simulink model "tb_FFT"  (R2024a)
settings: Solver=FixedStepDiscrete  StartTime=0.0  StopTime=400  RelTol=1e-3
undefined symbols (not defined in the file): F1, F2, FFTLength, Fs, ReadyIn, Reset, TestMode, Threshold
libraries: dsphdlxfrm2 x1, simulink x1
settings Model: DataTypeOverride=Off  Creator=bsingh  LastModifiedBy=bsingh
settings OptimizationCC: BlockReduction=off  ConditionallyExecuteInputs=off  DefaultParameterBehavior=Inlined  InheritOutputTypeSmallerThanSingle=on  OptimizeBlockIOStorage=off  ReuseModelBlockBuffer=off  EnhancedBackFolding=on  PassReuseOutputArgsThreshold=0  OptimizeBlockOrder=speed  DifferentSizesBufferReuse=on
settings DebuggingCC: AlgebraicLoopMsg=error  SingleTaskRateTransMsg=error  ParameterTunabilityLossMsg=error
settings HardwareCC: ProdBitPerPointer=32  ProdBitPerSizeT=32  ProdBitPerPtrDiffT=32  ProdLargestAtomicFloat=None  ProdIntDivRoundTo=Undefined  ProdEndianess=Unspecified  ProdWordSize=32  ProdHWDeviceType=ASIC/FPGA->ASIC/FPGA  TargetBitPerPointer=64  TargetBitPerSizeT=64  TargetBitPerPtrDiffT=64  TargetLongLongMode=on  TargetIntDivRoundTo=Zero  TargetEndianess=LittleEndian  TargetWordSize=64  TargetHWDeviceType=Generic->Custom  ProdEqTarget=off
settings SFSimCC: MATLABDynamicMemAllocThreshold=1024
settings RTWCC: Description=SystemVerilog DPI Component Generator  SystemTargetFile=systemverilog_dpi_grt.tlc  TemplateMakefile=systemverilog_dpi_grt_default_tmf  GPUComputeCapability=3.5
settings CodeAppCC: ForceParamTrailComments=on  MaxIdLength=256  OperatorAnnotations=on
settings DPIGRTTargetCC: TargetFcnLib=ansi_tfl_table_tmw.mat  GenFloatMathFcnCalls=NOT IN USE  TargetLangStandard=C89/C90 (ANSI)  CodeReplacementLibrary=None  UtilityFuncGeneration=Auto  MultiwordTypeDef=System defined  MultiwordLength=2048  DynamicStringBufferSize=256  GenerateFullHeader=on  InferredTypesCompatibility=off  GenerateSampleERTMain=off  GenerateTestInterfaces=off  ModelReferenceCompliant=on  ParMdlRefBuildCompliant=on  CompOptLevelCompliant=off  ConcurrentExecutionCompliant=off  IncludeMdlTerminateFcn=on  CombineOutputUpdateFcns=off  CombineSignalStateStructs=on  GroupInternalDataByFunction=off  SuppressErrorStatus=off  IncludeFileDelimiter=Auto  ERTCustomFileBanners=off  SupportAbsoluteTime=on  LogVarNameModifier=rt_  MatFileLogging=off  CodeInterfacePackaging=Reusable function  PurelyIntegerCode=off  SupportNonFinite=on  SupportComplex=on  SupportContinuousTime=on  SupportNonInlinedSFcns=on  RemoveDisableFunc=off  RemoveResetFunc=off  SupportVariableSizeSignals=off  ParenthesesLevel=Nominal  CastingMode=Nominal  MATLABClassNameForMDSCustomization=Simulink.SoftwareTarget.TargetSpecificTriggerConfigurationBase  ModelStepFunctionPrototypeControlCompliant=off  CPPClassGenCompliant=off  AutosarCompliant=off  MDXCompliant=off  GRTInterface=off  GenerateAllocFcn=on  UseToolchainInfoCompliant=on  GenerateSharedConstants=on  CoderGroups=[]  AccessMethods=[]  LookupTableObjectStructAxisOrder=1,2,3,4,...  LUTObjectStructOrderExplicitValues=Size,Breakpoints,Table  LUTObjectStructOrderEvenSpacing=Size,Breakpoints,Table  ArrayLayout=Column-major  UnsupportedSFcnMsg=error  ERTHeaderFileRootName=$R$E  ERTSourceFileRootName=$R$E  ERTDataFileRootName=$R_data  InstructionSetFMA=off  OptimizeReductions=off  LogToMDFFile=off  DPICustomizeSystemVerilogCode=off  DPISystemVerilogTemplate=svdpi_event.vgt  DPIReportRunTimeError=off  DPIRunTimeErrorSeverity=Fatal  DPIScalarizePorts=off  DPIGenerateTestBench=off  DPITestBenchSimulator=Mentor Graphics Questasim  DPITestPointAccessFcnInterface=None  DPIFixedPointDataType=CompatibleCType  DPIPortConnection=Port list  DPICompositeDataType=Structure  DPIComponentTemplateType=Sequential  ExtMode=off  ExtModeStaticAlloc=off  ExtModeTesting=off  ExtModeStaticAllocSize=1000000  ExtModeTransport=0  ExtModeMexFile=ext_comm  RTWCAPISignals=on  RTWCAPIParams=off  RTWCAPIStates=off  RTWCAPIRootIO=off  GenerateASAP2=off  MultiInstanceErrorCode=Error

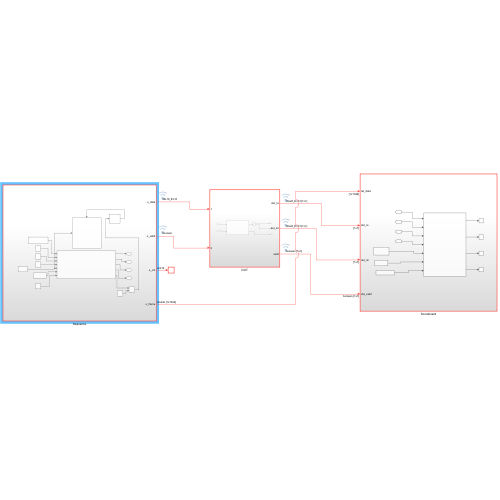
[thumbnail: Simulink's stored preview of the top-level diagram]
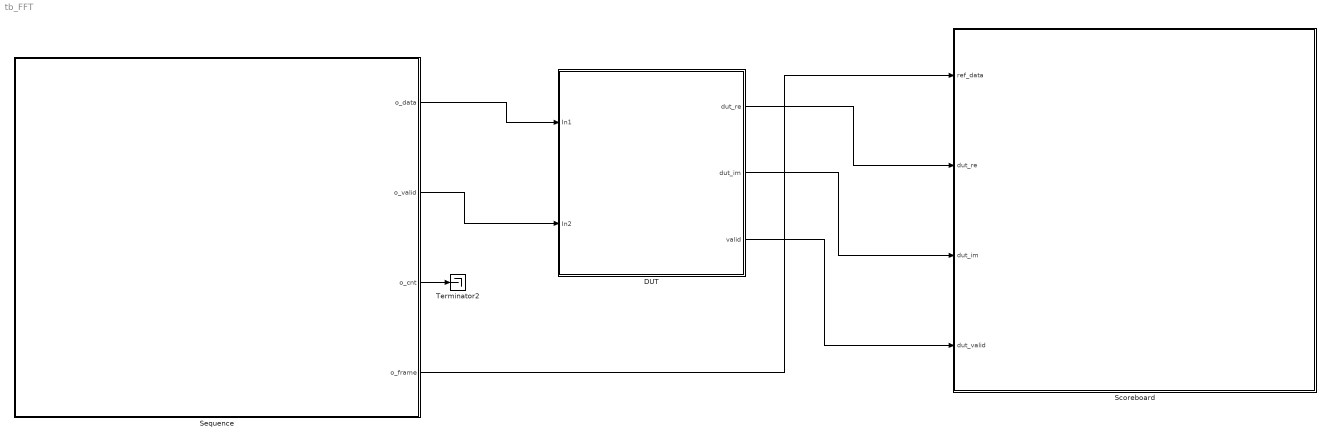
== system tb_FFT ==
  DUT : Subsystem
  Scoreboard : Subsystem
  Sequence : Subsystem
  Terminator2 : Terminator
  wires:
  Sequence/4(o_frame) -> Scoreboard/1(ref_data)
  Sequence/3(o_cnt) -> Terminator2/1
  Sequence/2(o_valid) -> DUT/2(In2)
  Sequence/1(o_data) -> DUT/1(In1)
  DUT/1(dut_re) -> Scoreboard/2(dut_re)
  DUT/2(dut_im) -> Scoreboard/3(dut_im)
  DUT/3(valid) -> Scoreboard/4(dut_valid)

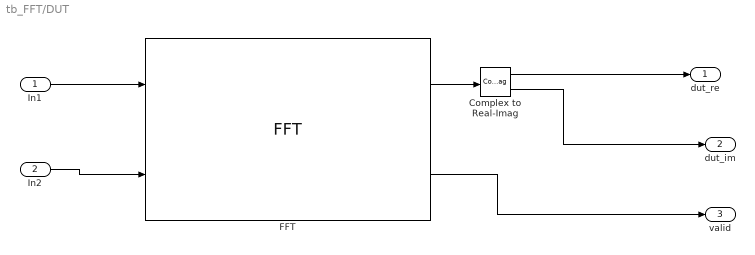
== system tb_FFT/DUT ==
  In1 : Inport
  In2 : Inport  Port=2
  Complex to Real-Imag : ComplexToRealImag
  FFT : dsphdlxfrm2/FFT  Architecture=Streaming Radix 2^2  FFTLengthSource=Property  FFTLength=DUT_FFTLength  FFTLengthMax=1024  ComplexMultiplication=Use 4 multipliers and 2 adders  BitReversedOutput=off  BitReversedInput=off  Normalize=off  SimulateUsing=Code generation  RoundingMethod=Floor  ResetInputPort=off  StartOutputPort=off  EndOutputPort=off
  dut_re : Outport
  dut_im : Outport  Port=2
  valid : Outport  Port=3
  wires:
  FFT/1 -> Complex to Real-Imag/1
  Complex to Real-Imag/2 -> dut_im/1
  Complex to Real-Imag/1 -> dut_re/1
  FFT/2 -> valid/1
  In1/1 -> FFT/1
  In2/1 -> FFT/2

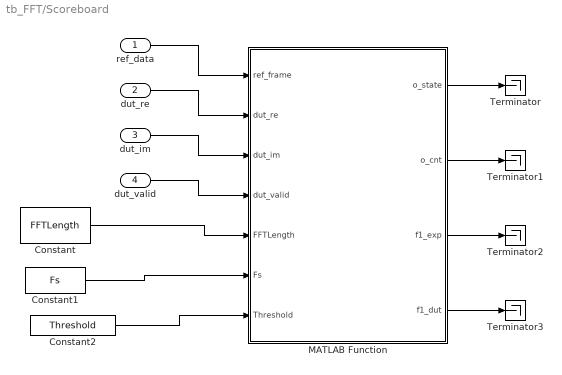
== system tb_FFT/Scoreboard ==
  ref_data : Inport
  dut_re : Inport  Port=2
  dut_im : Inport  Port=3
  dut_valid : Inport  Port=4  OutDataTypeStr=boolean
  Constant : Constant  Value=FFTLength  OutDataTypeStr=Inherit: Inherit via back propagation
  Constant1 : Constant  Value=Fs
  Constant2 : Constant  Value=Threshold
  MATLAB Function : MATLAB Function  TreatAsAtomicUnit=on
  Terminator{,1..3} (4 alike) : Terminator
  wires:
  ref_data/1 -> MATLAB Function/1(ref_frame)
  dut_re/1 -> MATLAB Function/2(dut_re)
  Constant1/1 -> MATLAB Function/6(Fs)
  Constant/1 -> MATLAB Function/5(FFTLength)
  dut_im/1 -> MATLAB Function/3(dut_im)
  dut_valid/1 -> MATLAB Function/4(dut_valid)
  Constant2/1 -> MATLAB Function/7(Threshold)
  MATLAB Function/1(o_state) -> Terminator/1
  MATLAB Function/2(o_cnt) -> Terminator1/1
  MATLAB Function/3(f1_exp) -> Terminator2/1
  MATLAB Function/4(f1_dut) -> Terminator3/1

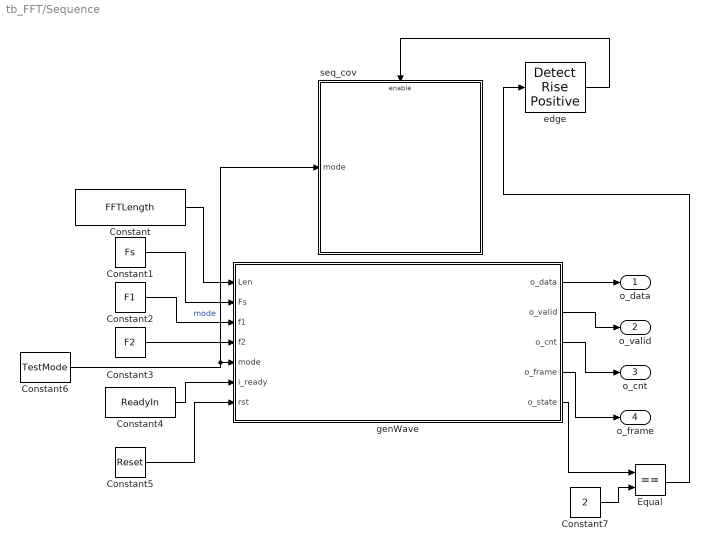
== system tb_FFT/Sequence ==
  Constant : Constant  Value=FFTLength
  Constant1 : Constant  Value=Fs  SampleTime=1e-1
  Constant2 : Constant  Value=F1
  Constant3 : Constant  Value=F2
  Constant4 : Constant  Value=ReadyIn
  Constant5 : Constant  Value=Reset
  Constant6 : Constant  Value=TestMode
  Constant7 : Constant  Value=2
  Equal : RelationalOperator  Operator===  OutDataTypeStr=boolean  RndMeth=Simplest  InputSameDT=off
  edge : simulink/Logic and Bit Operations/Detect Rise Positive  vinit=0  OutDataTypeStr=boolean
  genWave : MATLAB Function  TreatAsAtomicUnit=on
  seq_cov : Subsystem
  o_data : Outport
  o_valid : Outport  Port=2
  o_cnt : Outport  Port=3
  o_frame : Outport  Port=4
  wires:
  Constant5/1 -> genWave/7(rst)
  Constant4/1 -> genWave/6(i_ready)
  genWave/3(o_cnt) -> o_cnt/1
  Constant3/1 -> genWave/4(f2)
  Constant2/1 -> genWave/3(f1)
  Constant1/1 -> genWave/2(Fs)
  Constant/1 -> genWave/1(Len)
  genWave/1(o_data) -> o_data/1
  genWave/4(o_frame) -> o_frame/1
  genWave/2(o_valid) -> o_valid/1
  genWave/5(o_state) -> Equal/1
  Constant6/1 -> seq_cov/1(mode), genWave/5(mode)  "mode"
  Constant7/1 -> Equal/2
  Equal/1 -> edge/1
  edge/1 -> seq_cov/Enable

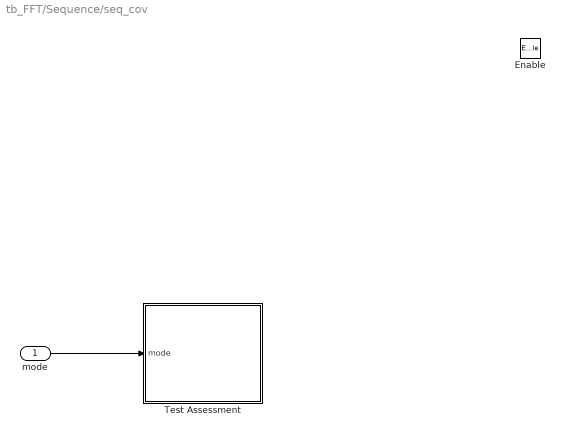
== system tb_FFT/Sequence/seq_cov ==
  mode : Inport
  Enable : EnablePort
  Test Assessment : Test Sequence  TreatAsAtomicUnit=on
  wires:
  mode/1 -> Test Assessment/1(mode)

== matlab function tb_FFT/Scoreboard/MATLAB Function ==
  data: ref_frame input; dut_re input; dut_im input; dut_valid input; FFTLength input; Fs input; o_state output; o_cnt output; Threshold input; f1_exp output; f1_dut output
function [o_state,o_cnt,f1_exp,f1_dut] = scbd(ref_frame,dut_re, dut_im,dut_valid,FFTLength, Fs,Threshold)

[o_state,o_cnt,f1_exp,f1_dut] = fftchecker(ref_frame,dut_re,dut_im,dut_valid,double(FFTLength),double(Fs),Threshold);

end

== matlab function tb_FFT/Sequence/genWave ==
  data: Len input; o_data output; Fs input; f1 input; f2 input; mode input; i_ready input; rst input; o_valid output; o_cnt output; o_frame output; o_state output
function [o_data,o_valid,o_cnt,o_frame,o_state] = genWave(Len,Fs,f1,f2,mode,i_ready,rst)%#codegen

[o_data,o_valid,o_cnt,o_frame,o_state] = genframe2Sample(Len, Fs,f1,f2,mode,i_ready,rst);

end

== stateflow chart tb_FFT/Sequence/seq_cov/Test Assessment ==
  state Assessments
    state verifyMode01
      verify(true, 'cg_mode:testmode_01', 'Verified Mode_01 in Simulation' )
    state verifyMode23
      verify(true,'cg_mode:testmode_23' ,'Verified Mode_23 in Simulation')
    state Else
    Assessments -> (junction 22)
    (default) -> (junction 22)
    (junction 22) -> (junction 23) [order 1] : [(mode <= 1)
        | ]
    (junction 23) -> verifyMode01 [order 1] : [~in(Assessments.verifyMode01)]
    (junction 22) -> (junction 31) [order 2]
    (junction 23) -> (junction 26) [order 2]
    (junction 31) -> (junction 32) [order 1] : [(mode > 1 && mode <=3)
        | ]
    (junction 32) -> verifyMode23 [order 1] : [~in(Assessments.verifyMode23)]
    (junction 32) -> (junction 35) [order 2]
    (junction 42) -> (junction 43)
    (junction 43) -> Else [order 1] : [~in(Assessments.Else)]
    (junction 43) -> (junction 46) [order 2]
    (junction 31) -> (junction 42) [order 2]
  (default) -> Assessments
  data: mode input
